simulink model "ex6"  (R2020b)
settings: Solver=VariableStepAuto  StartTime=0.0  StopTime=20  RelTol=1e-3
values from neighbouring files (symbols this model uses):
  den = [1 6 11.3223 18 12.81]    [ex6.m]    (also in ex6_control_2.m = [1 6 5+K 2*K*a K*a^2])
  num = [6.32 18 12.81]    [ex6.m]    (also in ex6_control_2.m = [K 2*K*a K*a^2])
libraries: cstblocks x2
settings Model: Creator=artur  LastModifiedBy=artur

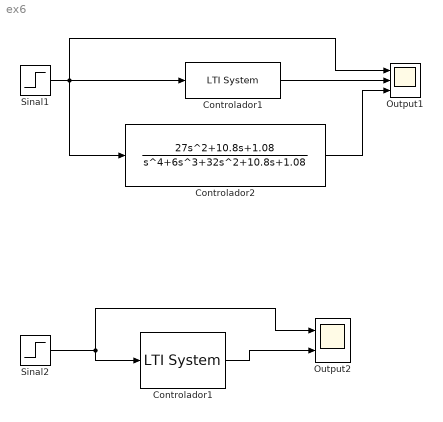
== system ex6 ==
  " Controlador1" : cstblocks/LTI System  sys=tf(num,den)  IC=[]
  Controlador1 : cstblocks/LTI System  sys=tf(num,den)  IC=[]
  Controlador2 : TransferFcn  Numerator=[27 10.8 1.08]  Denominator=[1 6 32 10.8 1.08]
  Output1 : Scope  NumInputPorts=3
  Output2 : Scope  NumInputPorts=2
  Sinal1 : Step  SampleTime=0
  Sinal2 : Step  SampleTime=0
  wires:
  " Controlador1"/1 -> Output2/2
  Sinal1/1 -> Controlador2/1, Controlador1/1, Output1/1
  Sinal2/1 -> Output2/1, " Controlador1"/1
  Controlador2/1 -> Output1/3
  Controlador1/1 -> Output1/2
